simulink model "untitled1"  (Simulink 7.7)
settings: Solver=ode45  StartTime=0.0  StopTime=10.0  RelTol=1e-3
settings Model: Creator=ali  LastModifiedBy=ali

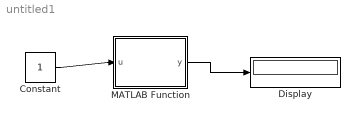
== system untitled1 ==
  Constant : Constant
  Display : Display
  MATLAB Function : Stateflow chart  TreatAsAtomicUnit=on
  wires:
  Constant/1 -> MATLAB Function/1(u)
  MATLAB Function/1(y) -> Display/1

== matlab function MATLAB Function ==
  data: u input double; y output double; nur_70_170 parameter double
function y = fcn(u, nur_70_170)
%#codegen

y = u+nur_70_170(5,2);
